simulink model "Vjezba3Z2"  (R2017a)
settings: Solver=VariableStepAuto  StartTime=0.0  StopTime=10.0  RelTol=1e-3
settings Model: Creator=korisnik  LastModifiedBy=korisnik

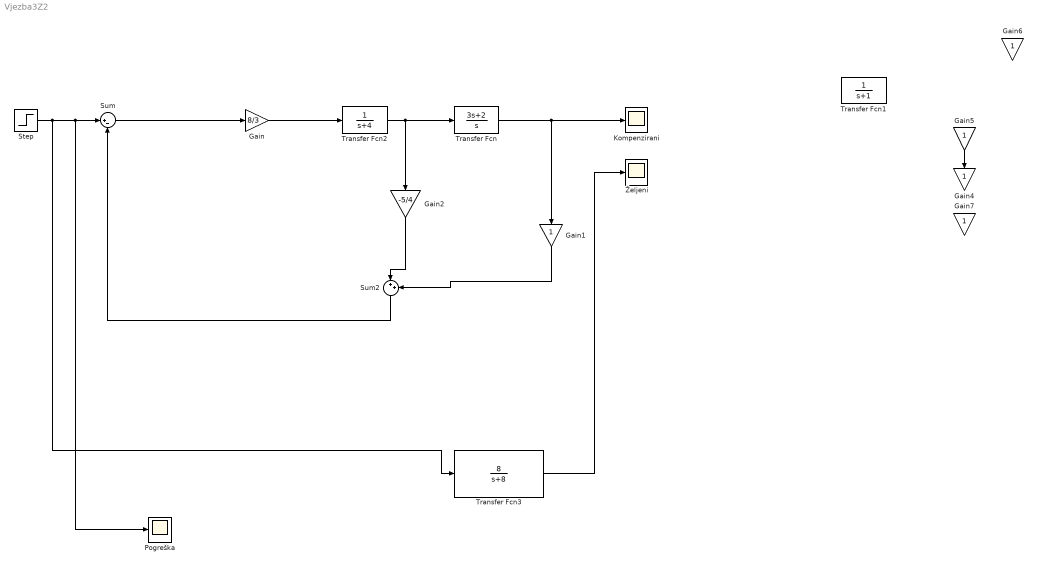
== system Vjezba3Z2 ==
  Gain : Gain  Gain=8/3
  Gain{1,4..7} (5 alike) : Gain
  Gain2 : Gain  Gain=-5/4
  Kompenzirani : Scope
  Pogreška : Scope
  Step : Step  SampleTime=0
  Sum : Sum  Inputs=|+-
  Sum2 : Sum  Inputs=|++
  Transfer Fcn : TransferFcn  Numerator=[3 2]  Denominator=[1 0]
  Transfer Fcn1 : TransferFcn  Denominator=[1 1]
  Transfer Fcn2 : TransferFcn  Denominator=[1 4]
  Transfer Fcn3 : TransferFcn  Numerator=[8]  Denominator=[1 8]
  Željeni : Scope
  wires:
  Step/1 -> Transfer Fcn3/1, Pogreška/1, Sum/1
  Sum/1 -> Gain/1
  Transfer Fcn2/1 -> Transfer Fcn/1, Gain2/1
  Transfer Fcn/1 -> Kompenzirani/1, Gain1/1
  Gain2/1 -> Sum2/1
  Gain1/1 -> Sum2/2
  Sum2/1 -> Sum/2
  Gain5/1 -> Gain4/1
  Transfer Fcn3/1 -> Željeni/1
  Gain/1 -> Transfer Fcn2/1
